simulink model "hw1"  (R2020b)
settings: Solver=FixedStepAuto  StartTime=0.0  StopTime=10  FixedStep=0.0001  RelTol=1e-3
model workspace (MAT data in the model file):
  Analog_Amplitude = 1
  Analog_Frequncy = 1
libraries: simulink x1
settings Model: EnablePacing=on  Creator=max  LastModifiedBy=spraychamber

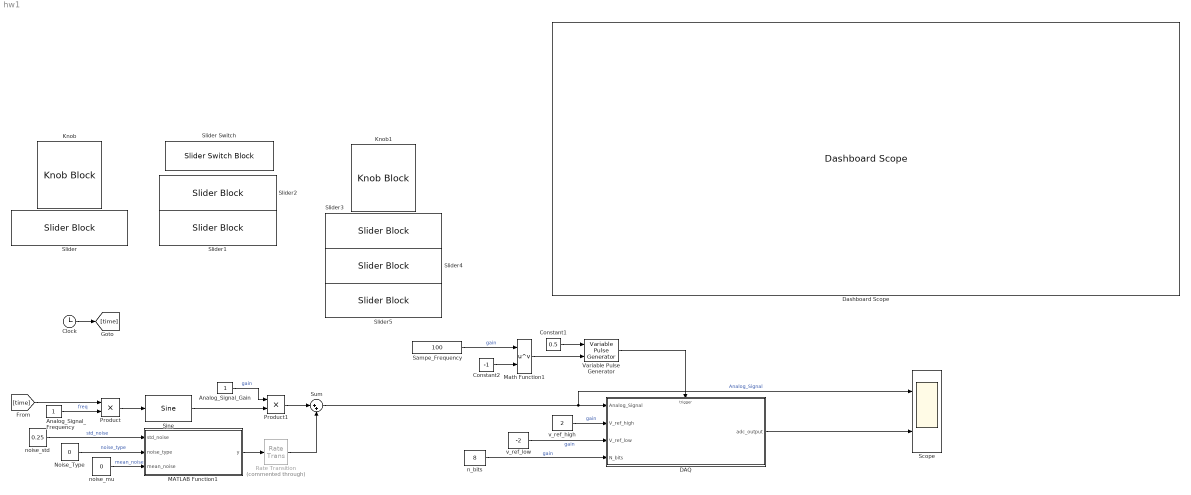
== system hw1 ==
  Analog_Signal_Frequency : Constant
  Analog_Signal_Gain : Constant
  Clock : Clock
  Constant1 : Constant  Value=0.5
  Constant2 : Constant  Value=-1
  DAQ : Subsystem
  Dashboard Scope : DashboardScope  Ymin=-10  Ymax=10
  Knob : KnobBlock  ScaleMin=1  ScaleMax=10000  ScaleType=Log
  Knob1 : KnobBlock  ScaleMin=1  ScaleMax=10000  ScaleType=Log
  MATLAB Function1 : MATLAB Function  TreatAsAtomicUnit=on
  Math Function1 : Math  Operator=pow  SaturateOnIntegerOverflow=on
  Noise_Type : Constant  Value=0
  Product : Product
  Product1 : Product
  Rate Transition : RateTransition  Commented=through  OutPortSampleTime=0.008
  Sampe_Frequency : Constant  Value=100
  Scope : Scope  NumInputPorts=2
  Sine : simulink/Lookup Tables/Sine  Formula=sin(2*pi*u)  NumDataPoints=(2^5)+1  OutputWordLength=16  InternalRulePriority=Speed
  Slider : SliderBlock  ScaleMax=10
  Slider Switch : SliderSwitchBlock
      settings: Values={{'Gaussian Noise', 'Uniform Noise'}, [0 1]}
  Slider1 : SliderBlock  ScaleMax=.5
  Slider2 : SliderBlock  ScaleMax=1
  Slider3 : SliderBlock  ScaleMax=10
  Slider4 : SliderBlock  ScaleMin=-10  ScaleMax=0
  Slider5 : SliderBlock  ScaleMax=10
  Sum : Sum  Inputs=|++
  Variable Pulse Generator : VariablePulseGenerator  RunAtFixedTimeIntervals=on  SampleTime=0.0001
  n_bits : Constant  Value=8
  noise_mu : Constant  Value=0
  noise_std : Constant  Value=0.25
  v_ref_high : Constant  Value=2
  v_ref_low : Constant  Value=-2
  wires:
  Clock/1 -> [time]
  Product/1 -> Sine/1
  Analog_Signal_Frequency/1 -> Product/2  "freq"
  Noise_Type/1 -> MATLAB Function1/2(noise_type)  "noise_type"
  noise_mu/1 -> MATLAB Function1/3(mean_noise)  "mean_noise"
  noise_std/1 -> MATLAB Function1/1(std_noise)  "std_noise"
  Analog_Signal_Gain/1 -> Product1/1  "gain"
  Sine/1 -> Product1/2
  Product1/1 -> Sum/1
  MATLAB Function1/1(y) -> Rate Transition/1
  Sum/1 -> Scope/1, DAQ/1(Analog_Signal)  "Analog_Signal"
  [time] -> Product/1
  DAQ/1(adc_output) -> Scope/2
  v_ref_low/1 -> DAQ/3(V_ref_low)  "gain"
  v_ref_high/1 -> DAQ/2(V_ref_high)  "gain"
  n_bits/1 -> DAQ/4(N_bits)  "gain"
  Constant2/1 -> Math Function1/2
  Math Function1/1 -> Variable Pulse Generator/2
  Constant1/1 -> Variable Pulse Generator/1
  Sampe_Frequency/1 -> Math Function1/1  "gain"
  Variable Pulse Generator/1 -> DAQ/Trigger
  Rate Transition/1 -> Sum/2

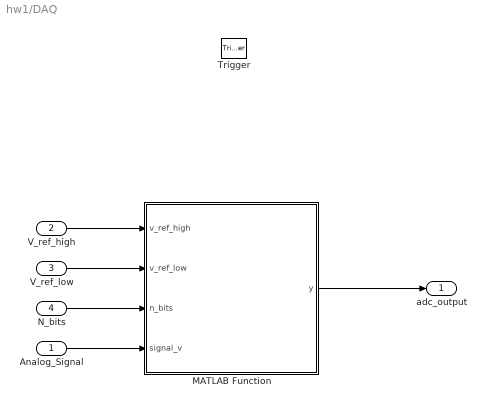
== system hw1/DAQ ==
  Analog_Signal : Inport
  V_ref_high : Inport  Port=2
  V_ref_low : Inport  Port=3
  N_bits : Inport  Port=4
  Trigger : TriggerPort  VariantControl=Variant  PortDimensions=1
  MATLAB Function : MATLAB Function  TreatAsAtomicUnit=on
  adc_output : Outport
  wires:
  V_ref_high/1 -> MATLAB Function/1(v_ref_high)
  V_ref_low/1 -> MATLAB Function/2(v_ref_low)
  Analog_Signal/1 -> MATLAB Function/4(signal_v)
  N_bits/1 -> MATLAB Function/3(n_bits)
  MATLAB Function/1(y) -> adc_output/1

== matlab function hw1/MATLAB Function1 ==
  data: y output; std_noise input; noise_type input; mean_noise input
function y = random_noise(std_noise, noise_type, mean_noise)
if noise_type == 0
    y = normrnd(mean_noise, std_noise);
else
    y = rand() * std_noise + mean_noise;
end

== matlab function hw1/DAQ/MATLAB Function ==
  data: v_ref_high input; y output; v_ref_low input; n_bits input; signal_v input
function y = daq(v_ref_high, v_ref_low, n_bits, signal_v)
v_ref_high = v_ref_high + abs(v_ref_low);
resolution = 2^n_bits;
delta = v_ref_high / resolution;
binary = zeros(resolution, 1);
signal_v = signal_v + abs(v_ref_low);
for i=1:resolution
    comparator = v_ref_high - i * delta;
    bit = signal_v >= comparator;
    binary(i) = (bit * comparator);
    if bit
        signal_v = signal_v - comparator;
    end
end
y = sum(binary) - abs(v_ref_low);
